simulink model "PMSM_FOC_Tractio"  (R2019b)
settings: Solver=FixedStepAuto  StartTime=0.0  StopTime=10  RelTol=1e-3
model workspace (MAT data in the model file):
  wc : Simulink.Parameter (value not decoded)
values from neighbouring files (symbols this model uses):
  CL_Param = tmp_CL_Param    [PMSM_Parameters.m]
  Cosine_table = [1,0.999995293095708,0.999990587122738,0.999985881149769,0.999981174245477,0.999967055395246,0.999952936545014,0.999938818626106,0.999924698844552,0.999901168979704,0.999877639114857,0.999854108318687,0.999830577522516,0.999797635711730,0.999764694832265,0.999731753021479,0.999698810279369,0.999656459316611,0.999614108353853,0.999571758322418,0.999529405497015,0.999477646313608,0.999425887130201,0 ...(+75635 chars)    [Motor_Table.m]
  ctrlParamsPI = tmp_ctrlParamsPI    [PMSM_Parameters.m]
  Flux_weak = tmp_Fluxweak_struct    [PMSM_Parameters.m]
  Hall_Parameter = tmp_Hall_struct    [PMSM_Parameters.m]
  HFI = tmp_HFI_struct    [PMSM_Parameters.m]
  inverter = struct    [PMSM_Parameters.m]
  MTPA_id_table = [-1.39452500000000,-1.36697494250000,-1.33970177000000,-1.31270548250000,-1.28598608000000,-1.25954356250000,-1.23337793000000,-1.20748918250000,-1.18187732000000,-1.15654234250000,-1.13148425000000,-1.10670304250000,-1.08219872000000,-1.05797128250000,-1.03402073000000,-1.01034706250000,-0.986950280000000,-0.963830382500000,-0.940987370000000,-0.918421242500000,-0.896132000000000,-0.8741196425000 ...(+3439 chars)    [Motor_Table.m]
  MTPA_iq_table = [-10.2740250000000,-10.1791705677750,-10.0840783722000,-9.98875081492500,-9.89319029760000,-9.79739922187500,-9.70137998940000,-9.60513500182500,-9.50866666080000,-9.41197736797500,-9.31506952500000,-9.21794553352500,-9.12060779520000,-9.02305871167500,-8.92530068460000,-8.82733611562500,-8.72916740640000,-8.63079695857500,-8.53222717380000,-8.43346045372500,-8.33449920000000,-8.23534581427500,-8. ...(+3121 chars)    [Motor_Table.m]
  MTPA_Te_Max = single(1.50)    [Motor_Table.m]
  MTPA_Te_Min = single(-1.50)    [Motor_Table.m]
  OPL_Param = tmp_OPL_Param    [PMSM_Parameters.m]
  pmsm = struct    [PMSM_Parameters.m]
  Resolver_Parameter = tmp_Resolver_struct    [PMSM_Parameters.m]
  Sine_table = [0,0.00153398793190718,0.00306797679513693,0.00460196565836668,0.00613595545291901,0.00766988657414913,0.00920381769537926,0.0107377488166094,0.0122716808691621,0.0138054965063930,0.0153393121436238,0.0168731296434999,0.0184069443494082,0.0199405867606401,0.0214742291718721,0.0230078706517816,0.0245415139943361,0.0260749254375696,0.0276083368808031,0.0291417483240366,0.0306751597672701,0.032208281 ...(+75648 chars)    [Motor_Table.m]
  SMO = temp_SMO    [PMSM_Parameters.m]
undefined symbols (not defined in the file or in its folder): DiscIntNeverNeededParam, Kiv, Kiw, Kpv, Kpw, magnitude, sigbuilder_block, SVPWM, Vdc
libraries: powerlib x29, fl_lib x18, simulink x10, nesl_utility x7, eeGeneralControl x4, dspstat3 x3, eeDiscretePi x2, powerlib_extras x1, ee_lib x1
(part 3 of 6)

== system PMSM_FOC_Tractio/Motor_Control/Motor_Control_Funtion/Angle_Speed_100us/Speed_Angle_Selector ==
  Resolver_Speed : Inport
  Resolver_Angle : Inport  Port=2
  Resolver_PLL_Speed : Inport  Port=3
  Resolver_PLL_Angle : Inport  Port=4
  Sensorless_Speed : Inport  Port=5
  Sensorless_Angle : Inport  Port=6
  Hall_Speed : Inport  Port=7
  Hall_Angle : Inport  Port=8
  Hall : Subsystem
  Hall_Angle_Enable : Constant  Value=Hall_Parameter.Angle_Enable  OutDataTypeStr=uint8
  If{1..3,5} (4 alike) : If  IfExpression=u1==1  ShowElse=off
  Merge : Merge  Inputs=4
  Merge1 : Merge  Inputs=4
  Resolver_Dir : Subsystem
  Resolver_Enable : Constant  Value=Resolver_Parameter.Angle_Enable  OutDataTypeStr=uint8
  Resolver_PLL : Subsystem
  Resolver_PLL_Enable : Constant  Value=Resolver_Parameter.PLL_Angle_Enable  OutDataTypeStr=uint8
  Sensorless : Subsystem
  Sensorless_Enable : Constant  Value=OPL_Param.Func_Enable  OutDataTypeStr=uint8
  Speed : Outport
  Theta : Outport  Port=2
  wires:
  If5/1 -> Resolver_Dir/Action
  Resolver_Enable/1 -> If5/1
  Hall_Speed/1 -> Hall/1(In1)
  Hall_Angle/1 -> Hall/2(In2)
  Sensorless_Speed/1 -> Sensorless/1(In1)
  Sensorless_Angle/1 -> Sensorless/2(In2)
  Resolver_Speed/1 -> Resolver_Dir/1(In1)
  Resolver_Angle/1 -> Resolver_Dir/2(In2)
  Resolver_PLL_Speed/1 -> Resolver_PLL/1(In1)
  Resolver_PLL_Angle/1 -> Resolver_PLL/2(In2)
  If1/1 -> Resolver_PLL/Action
  Resolver_PLL_Enable/1 -> If1/1
  Sensorless_Enable/1 -> If2/1
  If2/1 -> Sensorless/Action
  Hall_Angle_Enable/1 -> If3/1
  If3/1 -> Hall/Action
  Resolver_Dir/1(Out1) -> Merge/1
  Resolver_PLL/1(Out1) -> Merge/2
  Sensorless/1(Out1) -> Merge/3
  Hall/1(Out1) -> Merge/4
  Resolver_Dir/2(Out2) -> Merge1/1
  Resolver_PLL/2(Out2) -> Merge1/2
  Sensorless/2(Out2) -> Merge1/3
  Hall/2(Out2) -> Merge1/4
  Merge1/1 -> Theta/1
  Merge/1 -> Speed/1

== system PMSM_FOC_Tractio/Motor_Control/Motor_Control_Funtion/Angle_Speed_100us/Speed_Resolver ==
  Theta : Inport
  Action Port : ActionPort  ActionPortLabel=if(u1==1)
  DT2 : DataTypeConversion  OutDataTypeStr=single
  Scope : Scope
  Scope1 : Scope
  Speed_cacl : Subsystem  TreatAsAtomicUnit=on
      settings: RTWSystemCode=Nonreusable function  RTWFcnNameOpts=Use subsystem name
  Speed_out : Outport
  Dir_Angle : Outport  Port=2
  wires:
  Theta/1 -> DT2/1, Speed_cacl/1(position)  "Theta_input"
  Speed_cacl/1(Speed_RPM) -> Scope1/1, Speed_out/1  "Speed_RPM_Filtered"
  DT2/1 -> Scope/1, Dir_Angle/1  "Direct_Angle"

== system PMSM_FOC_Tractio/Motor_Control/Motor_Control_Funtion/Angle_Speed_100us/Startup_OPL ==
  OPL_Torque : Inport
  OPL_State : Inport  Port=2
  Smo_theta : Inport  Port=3
  Action Port : ActionPort  ActionPortLabel=if(u1==2|u1==3 | u1==3)
  If2 : If  IfExpression=u1==2  ElseIfExpressions=u1==3  ShowElse=off
  Merge : Merge
  Merge1 : Merge
  OPL_SpeedRPM : Constant  Value=OPL_Param.Target_RPM
  Scope3 : Scope  NumInputPorts=3
  Subsystem : Subsystem
  Subsystem1 : Subsystem
  Force_Angle : Outport
  OPL_Torque_Com : Outport  Port=2
  wires:
  OPL_State/1 -> If2/1
  If2/1 -> Subsystem/Action
  OPL_Torque/1 -> Subsystem1/1(OPL_Torque), Subsystem/2(OPL_Torque)
  If2/2 -> Subsystem1/Action
  Subsystem/1(Force_Angle) -> Merge/1
  Subsystem1/1(Force_Angle) -> Merge/2
  Merge/1 -> Force_Angle/1  "FOC_Angle"
  Subsystem/2(OPL_Torque_Com) -> Merge1/1
  Subsystem1/2(OPL_Torque_Com) -> Merge1/2
  Merge1/1 -> OPL_Torque_Com/1  "FOC_Angle"
  OPL_SpeedRPM/1 -> Subsystem1/3(Force_RPM), Subsystem/1(OPL_Speed)
  Smo_theta/1 -> Scope3/2, Subsystem/3(Smo_theta)
  Subsystem/3(Delta_theta) -> Subsystem1/2(Delta_theta)
  Subsystem/4(Force_Switch) -> Scope3/3, Subsystem1/4(Force_Switch)
  Subsystem1/3(Force_Angle1) -> Scope3/1

== system PMSM_FOC_Tractio/Motor_Control/Motor_Control_Funtion/Angle_Speed_100us/Subsystem ==
  Action Port : ActionPort  ActionPortLabel=if((u1==1)&(u2==1))
  Sensorless_Enable : Constant  OutDataTypeStr=boolean
  Out1 : Outport
  wires:
  Sensorless_Enable/1 -> Out1/1

== system PMSM_FOC_Tractio/Motor_Control/Motor_Control_Funtion/Angle_Speed_100us/Subsystem1 ==
  Action Port : ActionPort  ActionPortLabel=else
  Sensorless_Disable : Constant  Value=0  OutDataTypeStr=boolean
  Out1 : Outport
  wires:
  Sensorless_Disable/1 -> Out1/1

== system PMSM_FOC_Tractio/Motor_Control/Motor_Control_Funtion/Control_Command_2ms/Speed_PI ==
  Speed_Command : Inport
  Speed_Measured : Inport  Port=2
  HFI_State : Inport  Port=3
  Motor_State : Inport  Port=4
  BLDC_State : Inport  Port=5
  Action Port : ActionPort  ActionPortLabel=case [ 1 ]:
  Add2 : Sum  Inputs=|+-
  Hall_Enalble : Constant  Value=Hall_Parameter.BLDC_Start  OutDataTypeStr=uint8
  If1 : If  NumInputs=2  IfExpression=(u1==1)&(u2==3)|(u1~=1)  ShowElse=off
  Scope2 : Scope
  Speed_PI : Subsystem
  Iq_ref : Outport  VectorParamsAs1DForOutWhenUnconnected=off
  wires:
  Speed_Command/1 -> Add2/1
  Speed_Measured/1 -> Add2/2
  Add2/1 -> Speed_PI/1(PI_input)  "currentControlError"
  Speed_PI/1(PI_out) -> Iq_ref/1, Scope2/1
  HFI_State/1 -> Speed_PI/2(HFI_State)
  Motor_State/1 -> Speed_PI/3(Motor_State)
  BLDC_State/1 -> If1/2
  Hall_Enalble/1 -> If1/1
  If1/1 -> Speed_PI/Action

== system PMSM_FOC_Tractio/Motor_Control/Motor_Control_Funtion/Control_Command_2ms/Switch Case Action Subsystem ==
  Iq_in : Inport
  Action Port : ActionPort  ActionPortLabel=case [ 2 ]:
  Iq_out : Outport
  wires:
  Iq_in/1 -> Iq_out/1

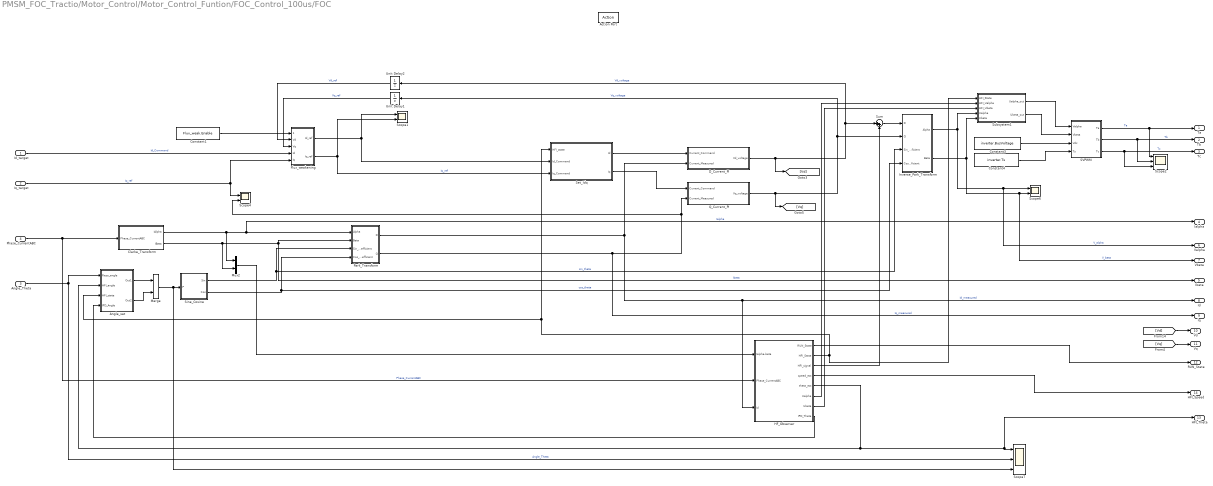
== system PMSM_FOC_Tractio/Motor_Control/Motor_Control_Funtion/FOC_Control_100us/FOC ==
  Id_target : Inport
  Iq_target : Inport  Port=2
  Angle_Theta : Inport  Port=3  OutMin=0  OutMax=2*pi
  Phase_CurrentABC : Inport  Port=4  PortDimensions=3
  Action Port : ActionPort  ActionPortLabel=if((u1==1)&(u2==3)|(u1~=1))
  Angle_set : Subsystem  TreatAsAtomicUnit=on
      settings: RTWSystemCode=Nonreusable function  RTWFcnNameOpts=Use subsystem name
  Clarke_Transform : Subsystem  TreatAsAtomicUnit=on
      settings: RTWSystemCode=Nonreusable function  RTWFcnNameOpts=Use subsystem name
  Constant1 : Constant  Value=Flux_weak.Enable  OutDataTypeStr=single
  Constant3 : Constant  Value=inverter.BusVoltage  OutDataTypeStr=single
  Constant4 : Constant  Value=inverter.Ts  OutDataTypeStr=single
  D_Current_PI : Subsystem  TreatAsAtomicUnit=on
      settings: RTWSystemCode=Nonreusable function  RTWFcnNameOpts=Use subsystem name
  "Flux_weakening " : Subsystem
  HF_Observer : Subsystem  TreatAsAtomicUnit=on
      settings: RTWSystemCode=Nonreusable function  RTWFcnNameOpts=Use subsystem name  RTWFileNameOpts=Use subsystem name
  Inverse_Park_Transform : Subsystem  TreatAsAtomicUnit=on
      settings: RTWSystemCode=Nonreusable function  RTWFcnNameOpts=Use subsystem name
      mask Display:
      | port_label('input',1,'D')
      | port_label('input',2,'Q')
      | port_label('input',3,'Sin')
      | port_label('input',4,'Cos')
      | port_label('output',1,'\alpha','texmode', 'on')
      | port_label('output',2,'\beta','texmode', 'on')
  Merge : Merge
  Mux2 : Mux  Inputs=2
  Park_Transform : Subsystem  TreatAsAtomicUnit=on
      settings: RTWSystemCode=Nonreusable function  RTWFcnNameOpts=Use subsystem name
      mask Display:
      | port_label('input',1,'\alpha','texmode', 'on')
      | port_label('input',2,'\beta','texmode', 'on')
      | port_label('input',3,'Sin')
      | port_label('input',4,'Cos')
      | port_label('output',1,'D')
      | port_label('output',2,'Q')
  Q_Current_PI : Subsystem  TreatAsAtomicUnit=on
      settings: RTWSystemCode=Nonreusable function  RTWFcnNameOpts=Use subsystem name
  SVPWM : Subsystem  AncestorBlock=SVPWM/SVPWM  TreatAsAtomicUnit=on  RTWFcnName=SVPWM  RTWFileName=SVPWM
      settings: RTWSystemCode=Nonreusable function  RTWFcnNameOpts=Use subsystem name
      mask Display:
      | plot([0.000 0.020 0.041 0.061 0.082 0.102 0.122 0.143 0.163 0.184 0.204 0.224 0.245 0.265 0.286 0.306 0.327 0.347 0.367 0.388 0.408 0.429 0.449 0.469 0.490 0.510 0.531 0.551 0.571 0.592 0.612 0.633 0.653 0.673 0.694 0.714 0.735 0.755 0.776 0.796 0.816 0.837 0.857 0.878 0.898 0.918 0.939 0.959 0.980 1.000 ], ...
      |      [0.500 0.586 0.671 0.753 0.831 0.858 0.875 0.885 0.890 0.887 0.879 0.864 0.844 0.855 0.872 0.884 0.889 0.888 0.881 0.867 0.847 0.793 0.713 0.629 0.543 0.457 0.371 0.287 0.207 0.153 0.133 0.119 0.112 0.111 0.116 0.128 0.145 0.156 0.136 0.121 0.113 0.110 0.115 0.125 0.142 0.169 0.247 0.329 0.414 0.500 ])
  Scope1 : Scope  NumInputPorts=2
  Scope2 : Scope  NumInputPorts=3
  Scope4 : Scope  NumInputPorts=2
  Scope6 : Scope  NumInputPorts=2
  Scope7 : Scope  NumInputPorts=3
  Set_Idq : Subsystem  TreatAsAtomicUnit=on
      settings: RTWSystemCode=Nonreusable function  RTWFcnNameOpts=Use subsystem name
  Sine_Cosine : Subsystem  TreatAsAtomicUnit=on
      settings: RTWSystemCode=Nonreusable function  RTWFcnNameOpts=Use subsystem name
  Subsystem1 : Subsystem
  Sum : Sum  Inputs=|++
  Unit Delay1 : UnitDelay  SampleTime=-1  HasFrameUpgradeWarning=on
  Unit Delay2 : UnitDelay  SampleTime=-1  HasFrameUpgradeWarning=on
  Ta : Outport
  Tb : Outport  Port=2
  Tc : Outport  Port=3
  Ialpha : Outport  Port=4
  Ibeta : Outport  Port=5
  Valpha : Outport  Port=6
  Vbeta : Outport  Port=7
  Id : Outport  Port=8
  Iq : Outport  Port=9
  Vd : Outport  Port=10
  Vq : Outport  Port=11
  RUN_State : Outport  Port=12
  HFI_Theta : Outport  Port=13
  HFI_Speed : Outport  Port=14
  wires:
  Park_Transform/1(D) -> HF_Observer/3(Id), Id/1, D_Current_PI/2(Current_Measured)  "Id_measured"
  Constant4/1 -> SVPWM/4(Ts)
  SVPWM/3(Tc) -> Tc/1, Scope2/3  "Tc"
  SVPWM/2(Tb) -> Scope2/2, Tb/1  "Tb"
  Park_Transform/2(Q) -> Iq/1, Scope4/2, Q_Current_PI/2(Current_Measured)  "Iq_measured"
  Sine_Cosine/2(Cos) -> Park_Transform/4(Cos_Coefficient), Inverse_Park_Transform/4(Cos_Coefficient)  "cos_theta"
  Sine_Cosine/1(Sin) -> Park_Transform/3(Sin_Coefficient), Inverse_Park_Transform/3(Sin_Coefficient)  "sin_theta"
  Constant3/1 -> SVPWM/3(Vdc)
  D_Current_PI/1(Vd_voltage) -> [Vd], Unit Delay2/1, Sum/1  "Vd_voltage"
  Q_Current_PI/1(Vq_voltage) -> [Vq], Unit Delay1/1, Inverse_Park_Transform/2(Q)  "Vq_voltage"
  SVPWM/1(Ta) -> Scope2/1, Ta/1  "Ta"
  Id_target/1 -> "Flux_weakening "/4(Id)  "Id_Command"
  Iq_target/1 -> "Flux_weakening "/5(Iq), Scope4/1  "Iq_ref"
  Clarke_Transform/2(IBeta) -> Mux2/2, Ibeta/1, Park_Transform/2(Beta)  "Ibeta"
  Clarke_Transform/1(IAlpha) -> Ialpha/1, Park_Transform/1(Alpha), Mux2/1  "Ialpha"
  Unit Delay2/1 -> "Flux_weakening "/2(Vd)  "Vd_ref"
  Unit Delay1/1 -> "Flux_weakening "/3(Vq)  "Vq_ref"
  "Flux_weakening "/1(Id_ref) -> Scope1/1, Set_Idq/2(Id_Command)
  "Flux_weakening "/2(Iq_ref) -> Set_Idq/3(Iq_Command), Scope1/2  "Iq_ref"
  Constant1/1 -> "Flux_weakening "/1(Enable)
  Inverse_Park_Transform/1(Alpha) -> Scope6/1, Valpha/1, Subsystem1/4(Ualpha)  "V_alpha"
  Inverse_Park_Transform/2(Beta) -> Scope6/2, Vbeta/1, Subsystem1/5(Ubeta)  "V_beta"
  Phase_CurrentABC/1 -> HF_Observer/2(Phase_CurrentABC), Clarke_Transform/1(Phase_CurrentABC)  "Phase_CurrentABC"
  Sum/1 -> Inverse_Park_Transform/1(D)
  HF_Observer/3(HFI_signal) -> Sum/2
  HF_Observer/4(speed_est) -> HFI_Speed/1
  Angle_Theta/1 -> Scope7/2, Angle_set/1(Reso_angle)  "Angle_Theta"
  Mux2/1 -> HF_Observer/1(Ialpha-beta)
  HF_Observer/5(theta_est) -> HFI_Theta/1, Scope7/1, Angle_set/2(HFI_angle)
  Merge/1 -> Scope7/3, Sine_Cosine/1(P)
  Angle_set/1(Out1) -> Merge/1
  Angle_set/2(Out2) -> Merge/2
  Subsystem1/1(Ualpha_out) -> SVPWM/1(Valpha)
  Subsystem1/2(Ubeta_out) -> SVPWM/2(Vbeta)
  HF_Observer/6(Ualpha) -> Subsystem1/2(HFI_Ualpha)
  HF_Observer/7(Ubeta) -> Subsystem1/3(HFI_Ubeta)
  HF_Observer/2(HFI_State) -> Subsystem1/1(HFI_State), Set_Idq/1(HFI_state), Angle_set/3(HFI_state)
  HF_Observer/1(RUN_State) -> RUN_State/1
  Set_Idq/1(Id) -> D_Current_PI/1(Current_Command)
  Set_Idq/2(Iq) -> Q_Current_PI/1(Current_Command)
  HF_Observer/8(IPD_Theta) -> Angle_set/4(IPD_Angle)
  [Vq] -> Vq/1
  [Vd] -> Vd/1

== system PMSM_FOC_Tractio/Motor_Control/Motor_Control_Funtion/FOC_Control_100us/Iq_selector ==
  Motor_state : Inport
  PI_IQ : Inport  Port=2
  OPL_IQ : Inport  Port=3
  If1 : If  IfExpression=u1 ==2 | u1 ==3
  Merge : Merge
  Subsystem : Subsystem
  Subsystem1 : Subsystem
  Iq_ref : Outport
  wires:
  Motor_state/1 -> If1/1
  If1/1 -> Subsystem/Action
  OPL_IQ/1 -> Subsystem/1(In1)
  PI_IQ/1 -> Subsystem1/1(In1)
  Subsystem/1(Out1) -> Merge/1
  Subsystem1/1(Out1) -> Merge/2
  Merge/1 -> Iq_ref/1
  If1/2 -> Subsystem1/Action

== system PMSM_FOC_Tractio/Motor_Control/Motor_Control_Funtion/FOC_Control_100us/MTPA ==
  Te_ref : Inport
  1-D Lookup Table4 : Lookup_n-D  NumberOfTableDimensions=1  LookupTableObject=''  BreakpointsForDimension1=single(linspace(MTPA_Te_Min,MTPA_Te_Max,length(MTPA_id_table)));  BreakpointsForDimension1FirstPoint=10  BreakpointsForDimension2FirstPoint=10  BreakpointsForDimension1Spacing=12  BreakpointsForDimension2Spacing=12  IndexSearchMethod=Evenly spaced points  Table=MTPA_id_table  InterpMethod=Flat  DiagnosticForOutOfRangeInput=Error  InternalRulePriority=Speed  RndMeth=Simplest  InputSameDT=on
  1-D Lookup Table5 : Lookup_n-D  NumberOfTableDimensions=1  LookupTableObject=''  BreakpointsForDimension1=single(linspace(MTPA_Te_Min,MTPA_Te_Max,length(MTPA_id_table)));  BreakpointsForDimension1FirstPoint=10  BreakpointsForDimension2FirstPoint=10  BreakpointsForDimension1Spacing=12  BreakpointsForDimension2Spacing=12  IndexSearchMethod=Evenly spaced points  Table=MTPA_iq_table  InterpMethod=Flat  DiagnosticForOutOfRangeInput=Error  InternalRulePriority=Speed  RndMeth=Simplest  InputSameDT=on
  Saturation : Saturate  UpperLimit=MTPA_Te_Max-0.01  LowerLimit=MTPA_Te_Min+0.01
  Saturation1 : Saturate  UpperLimit=MTPA_Te_Max-0.01  LowerLimit=MTPA_Te_Min+0.01
  Id_ref : Outport
  Iq_ref : Outport  Port=2
  wires:
  Te_ref/1 -> Saturation1/1, Saturation/1
  Saturation/1 -> 1-D Lookup Table4/1
  Saturation1/1 -> 1-D Lookup Table5/1
  1-D Lookup Table4/1 -> Id_ref/1
  1-D Lookup Table5/1 -> Iq_ref/1

== system PMSM_FOC_Tractio/Motor_Control/Motor_Control_Funtion/Motor_State_10ms/Power_Cacl ==
  Id : Inport
  Vd : Inport  Port=2
  Iq : Inport  Port=3
  Vq : Inport  Port=4
  Add : Sum
  Product : Product
  Product1 : Product
  Power : Outport
  wires:
  Id/1 -> Product/1
  Vd/1 -> Product/2
  Iq/1 -> Product1/1
  Vq/1 -> Product1/2
  Product/1 -> Add/1
  Product1/1 -> Add/2
  Add/1 -> Power/1

== system PMSM_FOC_Tractio/Motor_Control/Motor_Control_Funtion/Motor_State_10ms/Torque_Cacl ==
  Id : Inport
  Iq : Inport  Port=2
  Constant : Constant  Value=3/2  OutDataTypeStr=single
  Constant1 : Constant  Value=pmsm.PolePairs  OutDataTypeStr=single
  Constant2 : Constant  Value=pmsm.FluxLinkage  OutDataTypeStr=single
  Constant3 : Constant  Value=pmsm.InductanceLd  OutDataTypeStr=single
  Constant4 : Constant  Value=pmsm.InductanceLq  OutDataTypeStr=single
  Product{,1..4} (5 alike) : Product
  Subtract : Sum
  Subtract1 : Sum  Inputs=+-
  Torque : Outport
  wires:
  Constant1/1 -> Product/1
  Constant/1 -> Product/2
  Constant2/1 -> Product1/1
  Iq/1 -> Product1/2, Product3/1
  Product1/1 -> Subtract/1
  Constant3/1 -> Subtract1/1
  Constant4/1 -> Subtract1/2
  Subtract1/1 -> Product2/1
  Id/1 -> Product2/2
  Product2/1 -> Product3/2
  Product3/1 -> Subtract/2
  Product/1 -> Product4/1
  Subtract/1 -> Product4/2
  Product4/1 -> Torque/1

== system PMSM_FOC_Tractio/PMSM/Control/Control/Commutation ==
  Hall : Inport
  Bias : Bias  Bias=-1
  Bit concatenate : Subsystem
  Data Type Conversion : DataTypeConversion
  Direct Lookup Table (n-D)2 : LookupNDDirect  InputsSelectThisObjectFromTable=Vector  Table=[0 0 0 1 1 0;0 1 1 0 0 0;0 1 0 0 0 1;1 0 0 0 1 0;1 0 1 0 0 0;0 0 0 1 0 1]
  S : Outport  VectorParamsAs1DForOutWhenUnconnected=off
  wires:
  Hall/1 -> Bit concatenate/1(u)
  Bit concatenate/1(y) -> Data Type Conversion/1
  Direct Lookup Table (n-D)2/1 -> S/1
  Data Type Conversion/1 -> Bias/1
  Bias/1 -> Direct Lookup Table (n-D)2/1

== system PMSM_FOC_Tractio/PMSM/SpeedAndAngle/ACC_OMG/Six_point ==
  In1 : Inport
  Merge2 : Merge  Inputs=6
  Scope : Scope  NumInputPorts=2
  Sector_1 : Subsystem
  Sector_2 : Subsystem
  Sector_3 : Subsystem
  Sector_4 : Subsystem
  Sector_5 : Subsystem
  Sector_6 : Subsystem
  Switch Case2 : SwitchCase  CaseConditions={1,2,3,4,5,6}  ShowDefaultCase=off
  Out1 : Outport
  wires:
  Sector_4/1(Angle_0) -> Merge2/4
  Switch Case2/5 -> Sector_5/Action
  Sector_6/1(Angle_0) -> Merge2/6
  Sector_5/1(Angle_0) -> Merge2/5
  Switch Case2/6 -> Sector_6/Action
  Switch Case2/3 -> Sector_3/Action
  Switch Case2/4 -> Sector_4/Action
  Sector_1/1(Angle_0) -> Merge2/1
  Switch Case2/2 -> Sector_2/Action
  In1/1 -> Scope/1, Switch Case2/1
  Sector_3/1(Angle_0) -> Merge2/3
  Switch Case2/1 -> Sector_1/Action
  Sector_2/1(Angle_0) -> Merge2/2
  Merge2/1 -> Scope/2, Out1/1

== system PMSM_FOC_Tractio/PMSM/SpeedAndAngle/ADC_IRQ/HallAngle_calibration ==
  Angle_input : Inport
  Angle_offset : Constant  Value=SMO.Angle_offset
  If Action Subsystem1 : Subsystem  TreatAsAtomicUnit=on
  If Action Subsystem2 : Subsystem  TreatAsAtomicUnit=on
  If Action Subsystem3 : Subsystem  TreatAsAtomicUnit=on
  If1 : If  IfExpression=u1 > 6.283185307  ElseIfExpressions=u1<0
  Merge1 : Merge  Inputs=3
  Subtract1 : Sum
  Angle_output : Outport
  wires:
  Angle_input/1 -> Subtract1/1
  Angle_offset/1 -> Subtract1/2  "Control_ModeCommand"
  If1/1 -> If Action Subsystem2/Action
  If1/3 -> If Action Subsystem1/Action
  If Action Subsystem2/1(Out1) -> Merge1/1
  Subtract1/1 -> If Action Subsystem3/1(In1), If Action Subsystem1/1(In1), If Action Subsystem2/1(In1), If1/1
  If Action Subsystem1/1(Out1) -> Merge1/3
  If Action Subsystem3/1(Out1) -> Merge1/2
  If1/2 -> If Action Subsystem3/Action
  Merge1/1 -> Angle_output/1

== system PMSM_FOC_Tractio/Motor_Control/Motor_Control_Funtion/Angle_Speed_100us/Angle_Selector/Subsystem ==
  In1 : Inport
  Action Port : ActionPort  ActionPortLabel=if(u1 ==2 | u1 ==3)
  Out1 : Outport
  wires:
  In1/1 -> Out1/1

== system PMSM_FOC_Tractio/Motor_Control/Motor_Control_Funtion/Angle_Speed_100us/Angle_Selector/Subsystem1 ==
  In1 : Inport
  Action Port : ActionPort  ActionPortLabel=elseif(u1 ==4)
  Out1 : Outport
  wires:
  In1/1 -> Out1/1

== system PMSM_FOC_Tractio/Motor_Control/Motor_Control_Funtion/Angle_Speed_100us/Resolver_Observer/Angle_calibration ==
  Angle_input : Inport
  Angle_offset : Constant  Value=Resolver_Parameter.PLL_Angle_offset
  If Action Subsystem1 : Subsystem  TreatAsAtomicUnit=on
  If Action Subsystem2 : Subsystem  TreatAsAtomicUnit=on
  If Action Subsystem3 : Subsystem  TreatAsAtomicUnit=on
  If1 : If  IfExpression=u1 > 6.283185307  ElseIfExpressions=u1<0
  Merge1 : Merge  Inputs=3
  Subtract1 : Sum
  Angle_output : Outport
  wires:
  If1/2 -> If Action Subsystem3/Action
  If Action Subsystem1/1(Out1) -> Merge1/3
  If1/3 -> If Action Subsystem1/Action
  If Action Subsystem3/1(Out1) -> Merge1/2
  If Action Subsystem2/1(Out1) -> Merge1/1
  Subtract1/1 -> If Action Subsystem3/1(In1), If Action Subsystem1/1(In1), If Action Subsystem2/1(In1), If1/1
  If1/1 -> If Action Subsystem2/Action
  Angle_offset/1 -> Subtract1/2
  Angle_input/1 -> Subtract1/1
  Merge1/1 -> Angle_output/1

== system PMSM_FOC_Tractio/Motor_Control/Motor_Control_Funtion/Angle_Speed_100us/Resolver_Observer/Resolver_Angle_cacl ==
  Sin_Cos : Inport
  2*pi : Constant  Value=2*pi  OutDataTypeStr=single  SampleTime=-1
  B : Selector  IndexMode=Zero-based  InputPortWidth=2  IndexOptions=Index vector (dialog)  Indices=0  OutputSizes=1
  C : Selector  IndexMode=Zero-based  InputPortWidth=2  IndexOptions=Index vector (dialog)  Indices=1  OutputSizes=1
  Constant : Constant  OutDataTypeStr=single  SampleTime=-1
  Discrete-Time Integrator : DiscreteIntegrator  SampleTime=-1  ICPrevOutput=DiscIntNeverNeededParam  ICPrevScaledInput=DiscIntNeverNeededParam
  Gain : Gain  Gain=15/(2*pi)
  LPF : DiscreteFilter  Numerator=[0 0.04]  Denominator=[1 -0.96]
  Math Function : Math  Operator=mod  SaturateOnIntegerOverflow=on
  PID Controller : simulink/Continuous/PID Controller  Controller=PI  Form=Parallel  TimeDomain=Discrete-time  SampleTime=-1  IntegratorMethod=Forward Euler  FilterMethod=Forward Euler  ControllerParametersSource=internal  P=141  I=10000  D=0  UseFilter=off  N=100  TunerSelectOption=Transfer Function Based (PID Tuner App)  InitialConditionSource=internal  InitialConditionForIntegrator=0  InitialConditionForFilter=0  DifferentiatorICPrevScaledInput=0  ExternalReset=none  TrackingMode=off  Kt=1  LimitOutput=off  UpperSaturationLimit=inf  LowerSaturationLimit=-inf  LinearizeAsGain=on  AntiWindupMode=none  Kb=1  POutMin=[]  POutMax=[]  IOutMin=[]  IOutMax=[]  DOutMin=[]  DOutMax=[]  NOutMin=[]  NOutMax=[]  SumOutMin=[]  SumOutMax=[]  SaturationOutMin=[]  SaturationOutMax=[]  PParamMin=[]  PParamMax=[]  IParamMin=[]  IParamMax=[]  DParamMin=[]  DParamMax=[]  NParamMin=[]  NParamMax=[]  KbParamMin=[]  KbParamMax=[]  KtParamMin=[]  KtParamMax=[]  KbOutMin=[]  KbOutMax=[]  KtOutMin=[]  KtOutMax=[]  IntegratorOutMin=[]  IntegratorOutMax=[]  FilterOutMin=[]  FilterOutMax=[]  SumI1OutMin=[]  SumI1OutMax=[]  SumI2OutMin=[]  SumI2OutMax=[]  SumI3OutMin=[]  SumI3OutMax=[]  SumI4OutMin=[]  SumI4OutMax=[]  SumDOutMin=[]  SumDOutMax=[]  DifferentiatorOutMin=[]  DifferentiatorOutMax=[]  FilterDiffOutCoefMin=[]  FilterDiffOutCoefMax=[]  ReciprocalOutMin=[]  ReciprocalOutMax=[]  SumDenOutMin=[]  SumDenOutMax=[]  SumNumOutMin=[]  SumNumOutMax=[]  DivideOutMin=[]  DivideOutMax=[]  IntegratorContinuousStateAttributes=''  IntegratorStateMustResolveToSignalObject=off  IntegratorRTWStateStorageClass=Auto  FilterContinuousStateAttributes=''  FilterStateMustResolveToSignalObject=off  FilterRTWStateStorageClass=Auto  ParallelPVariant=InternalParameters  IdealPVariant=Disabled  IVariant=InternalParameters  DVariant=Disabled  IntegratorVariant=Discrete  SatVariant=Disabled  AWVariant=Passthrough  PCopyVariant=Disabled  TRVariant=Disabled  FdbkBlocksVariant=Forward  IdealPFdbkVariant=Disabled  SatFdbkVariant=Disabled  DerivativeFilterVariant=Disabled  NVariant=Disabled  NCopyVariant=Disabled_SignalSpec  FilterICVariant=Disabled  IntegratorICVariant=InternalICs  ExternalResetVariant=Disabled  TRSumVariant=Passthrough  SumFdbkVariant=Disabled  SumVariant=Sum_PI
  Product : Product  OutDataTypeStr=single
  Product{1..4} (4 alike) : Product
  Scope : Scope  NumInputPorts=2
  Scope{1,3..4,6..7} (5 alike) : Scope
  Scope2 : Scope  NumInputPorts=2
  Scope5 : Scope  NumInputPorts=2
  Sine_Cosine : Subsystem  TreatAsAtomicUnit=on
      settings: RTWSystemCode=Nonreusable function  RTWFcnNameOpts=Use subsystem name
  Sum1 : Sum  Inputs=-+
  Unit Delay4 : UnitDelay  SampleTime=-1  HasFrameUpgradeWarning=on
  constant : Constant  OutDataTypeStr=single
  "pole pairs " : Gain  OutDataTypeStr=single
  Velocity : Outport  VectorParamsAs1DForOutWhenUnconnected=off
  Angle : Outport  Port=2  VectorParamsAs1DForOutWhenUnconnected=off
  wires:
  Product2/1 -> Scope2/2, Product4/1
  Product4/1 -> Scope/2, Sum1/2
  Sin_Cos/1 -> C/1, B/1
  Unit Delay4/1 -> Product/2
  Sum1/1 -> PID Controller/1
  Product3/1 -> Scope/1, Sum1/1
  Constant/1 -> Product/1
  constant/1 -> Product2/1, Product1/1
  Product/1 -> Sine_Cosine/1(P)
  Sine_Cosine/1(Sin) -> Product1/2
  Product1/1 -> Scope2/1, Product3/2
  Math Function/1 -> Unit Delay4/1, Angle/1, Scope4/1  "Angle_Theta"
  Gain/1 -> LPF/1, Scope3/1  "Speed_RPM"
  Discrete-Time Integrator/1 -> Scope6/1, "pole pairs "/1
  "pole pairs "/1 -> Math Function/1
  PID Controller/1 -> Discrete-Time Integrator/1, Gain/1
  2*pi/1 -> Math Function/2
  B/1 -> Scope1/1, Product3/1, Scope5/2, Scope5/1  "Vx"
  C/1 -> Product4/2, Scope7/1  "Vy"
  LPF/1 -> Velocity/1
  Sine_Cosine/2(Cos) -> Product2/2

== system PMSM_FOC_Tractio/Motor_Control/Motor_Control_Funtion/Angle_Speed_100us/SMO/Angle_calibration ==
  Angle_input : Inport
  Angle_offset : Constant  Value=SMO.Angle_offset
  If Action Subsystem1 : Subsystem  TreatAsAtomicUnit=on
  If Action Subsystem2 : Subsystem  TreatAsAtomicUnit=on
  If Action Subsystem3 : Subsystem  TreatAsAtomicUnit=on
  If1 : If  IfExpression=u1 > 6.283185307  ElseIfExpressions=u1<0
  Merge1 : Merge  Inputs=3
  Subtract1 : Sum
  Angle_output : Outport
  wires:
  Angle_input/1 -> Subtract1/1
  Angle_offset/1 -> Subtract1/2  "Control_ModeCommand"
  If1/1 -> If Action Subsystem2/Action
  If1/3 -> If Action Subsystem1/Action
  If Action Subsystem2/1(Out1) -> Merge1/1
  Subtract1/1 -> If Action Subsystem3/1(In1), If Action Subsystem1/1(In1), If Action Subsystem2/1(In1), If1/1
  If Action Subsystem1/1(Out1) -> Merge1/3
  If Action Subsystem3/1(Out1) -> Merge1/2
  If1/2 -> If Action Subsystem3/Action
  Merge1/1 -> Angle_output/1

== system PMSM_FOC_Tractio/Motor_Control/Motor_Control_Funtion/Angle_Speed_100us/SMO/Delta_theta ==
  Est_theta : Inport
  Ealpha_est : Inport  Port=2
  Ebeta_est : Inport  Port=3
  Add : Sum
  Add1 : Sum
  Divide : Product  Inputs=*/
  Gain : Gain  Gain=-1
  Math Function : Math  Operator=magnitude^2  SignedPower=off  SaturateOnIntegerOverflow=on
  Math Function1 : Math  Operator=magnitude^2  SignedPower=off  SaturateOnIntegerOverflow=on
  Product : Product
  Product1 : Product
  Saturation : Saturate  UpperLimit=inf  LowerLimit=4.0
  Sine_Cosine : Subsystem  TreatAsAtomicUnit=on
      settings: RTWSystemCode=Nonreusable function  RTWFcnNameOpts=Use subsystem name
  Sqrt : Sqrt  SaturateOnIntegerOverflow=on
  delta_theta : Outport
  unit : Outport  Port=2
  wires:
  Est_theta/1 -> Sine_Cosine/1(P)
  Ealpha_est/1 -> Math Function/1, Product/2
  Sine_Cosine/1(Sin) -> Product1/1
  Ebeta_est/1 -> Math Function1/1, Product1/2
  Product/1 -> Add/1
  Product1/1 -> Add/2
  Add/1 -> Gain/1
  Math Function/1 -> Add1/1
  Math Function1/1 -> Add1/2
  Add1/1 -> Sqrt/1
  Sqrt/1 -> Saturation/1
  Gain/1 -> Divide/1
  Saturation/1 -> unit/1, Divide/2
  Divide/1 -> delta_theta/1
  Sine_Cosine/2(Cos) -> Product/1

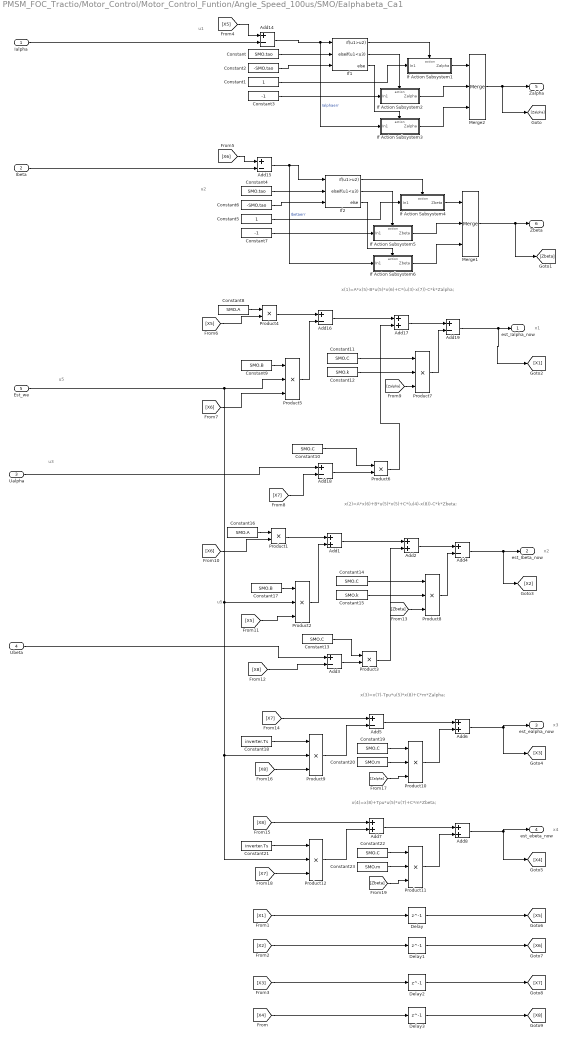
== system PMSM_FOC_Tractio/Motor_Control/Motor_Control_Funtion/Angle_Speed_100us/SMO/Ealphabeta_Ca1 ==
  note: x(4)=x(8)+Tpu*u(5)*x(7)+C*m*Zbeta;
  note: x(3)=x(7)-Tpu*u(5)*x(8)+C*m*Zalpha;
  note: x(2)=A*x(6)+B*u(5)*x(5)+C*(u(4)-x(8))-C*k*Zbeta;
  note: x(1)=A*x(5)-B*u(5)*x(6)+C*(u(3)-x(7))-C*k*Zalpha;
  note: x1
  note: u1
  note: u3
  note: u5
  note: u2
  note: u5
  note: x2
  note: x3
  note: x4
  Ialpha : Inport
  Ibeta : Inport  Port=2
  Ualpha : Inport  Port=3
  Ubeta : Inport  Port=4
  Est_we : Inport  Port=5
  Add{1..2,6..8,17} (6 alike) : Sum
  Add{3..5,14..16,18..19} (8 alike) : Sum  Inputs=+-
  Constant : Constant  Value=SMO.tao  OutDataTypeStr=single
  Constant1 : Constant  OutDataTypeStr=single
  Constant10 : Constant  Value=SMO.C  OutDataTypeStr=single
  Constant11 : Constant  Value=SMO.C  OutDataTypeStr=single
  Constant12 : Constant  Value=SMO.k  OutDataTypeStr=single
  Constant{13..14,19,22} (4 alike) : Constant  Value=SMO.C
  Constant15 : Constant  Value=SMO.k
  Constant16 : Constant  Value=SMO.A  OutDataTypeStr=single
  Constant17 : Constant  Value=SMO.B
  Constant18 : Constant  Value=inverter.Ts  OutDataTypeStr=single
  Constant2 : Constant  Value=-SMO.tao  OutDataTypeStr=single
  Constant20 : Constant  Value=SMO.m
  Constant21 : Constant  Value=inverter.Ts  OutDataTypeStr=single
  Constant23 : Constant  Value=SMO.m
  Constant3 : Constant  Value=-1  OutDataTypeStr=single
  Constant4 : Constant  Value=SMO.tao
  Constant5 : Constant  OutDataTypeStr=single
  Constant6 : Constant  Value=-SMO.tao
  Constant7 : Constant  Value=-1  OutDataTypeStr=single
  Constant8 : Constant  Value=SMO.A  OutDataTypeStr=single
  Constant9 : Constant  Value=SMO.B
  Delay{,1..3} (4 alike) : Delay  DelayLength=1  InitialCondition=0
  If Action Subsystem1 : Subsystem  TreatAsAtomicUnit=on
  If Action Subsystem2 : Subsystem  TreatAsAtomicUnit=on
  If Action Subsystem3 : Subsystem  TreatAsAtomicUnit=on
  If Action Subsystem4 : Subsystem  TreatAsAtomicUnit=on
  If Action Subsystem5 : Subsystem  TreatAsAtomicUnit=on
  If Action Subsystem6 : Subsystem  TreatAsAtomicUnit=on
  If1 : If  NumInputs=3  IfExpression=u1>u2  ElseIfExpressions=u1<u3
  If2 : If  NumInputs=3  IfExpression=u1>u2  ElseIfExpressions=u1<u3
  Merge1 : Merge  Inputs=3
  Merge2 : Merge  Inputs=3
  Product{1,3..4,6} (4 alike) : Product
  Product{2,5,7..12} (8 alike) : Product  Inputs=3
  est_Ialpha_now : Outport
  est_Ibeta_now : Outport  Port=2
  est_ealpha_now : Outport  Port=3
  est_ebeta_now : Outport  Port=4
  Zalpha : Outport  Port=5
  Zbeta : Outport  Port=6
  wires:
  Ialpha/1 -> Add14/2
  Add14/1 -> If Action Subsystem3/1(In1), If1/1  "Ialphaerr"
  Constant/1 -> If1/2
  If1/1 -> If Action Subsystem1/Action
  Constant1/1 -> If Action Subsystem1/1(In1)
  Constant3/1 -> If Action Subsystem2/1(In1)
  Constant2/1 -> If1/3
  If1/2 -> If Action Subsystem2/Action
  If1/3 -> If Action Subsystem3/Action
  If Action Subsystem1/1(Zalpha) -> Merge2/1
  If Action Subsystem2/1(Zalpha) -> Merge2/2
  If Action Subsystem3/1(Zalpha) -> Merge2/3
  Ibeta/1 -> Add15/2
  If2/1 -> If Action Subsystem4/Action
  If2/3 -> If Action Subsystem6/Action
  If Action Subsystem4/1(Zbeta) -> Merge1/1
  Constant5/1 -> If Action Subsystem4/1(In1)
  If2/2 -> If Action Subsystem5/Action
  Constant6/1 -> If2/3
  If Action Subsystem6/1(Zbeta) -> Merge1/3
  Constant7/1 -> If Action Subsystem5/1(In1)
  If Action Subsystem5/1(Zbeta) -> Merge1/2
  Add15/1 -> If2/1, If Action Subsystem6/1(In1)  "Ibetaerr"
  Constant4/1 -> If2/2
  Constant8/1 -> Product4/1
  Add19/1 -> [X1], est_Ialpha_now/1
  Product4/1 -> Add16/1
  Constant9/1 -> Product5/1
  Product5/1 -> Add16/2
  Add16/1 -> Add17/1
  Ualpha/1 -> Add18/1
  Add18/1 -> Product6/2
  Constant10/1 -> Product6/1
  Product6/1 -> Add17/2
  Add17/1 -> Add19/1
  Product7/1 -> Add19/2
  Constant11/1 -> Product7/1
  Constant12/1 -> Product7/2
  Product3/1 -> Add2/2
  Product8/1 -> Add4/2
  Constant15/1 -> Product8/2
  Constant16/1 -> Product1/1
  Add3/1 -> Product3/2
  Product2/1 -> Add1/2
  Add4/1 -> [X2], est_Ibeta_now/1
  Constant14/1 -> Product8/1
  Add1/1 -> Add2/1
  Constant13/1 -> Product3/1
  Ubeta/1 -> Add3/1
  Constant17/1 -> Product2/1
  Add2/1 -> Add4/1
  Product1/1 -> Add1/1
  Add6/1 -> est_ealpha_now/1, [X3]
  Constant18/1 -> Product9/1
  Product9/1 -> Add5/2
  Add5/1 -> Add6/1
  Constant19/1 -> Product10/1
  Constant20/1 -> Product10/2
  Product10/1 -> Add6/2
  Merge1/1 -> [Zbeta], Zbeta/1
  Constant21/1 -> Product12/1
  Constant22/1 -> Product11/1
  Est_we/1 -> Product12/2, Product9/2, Product2/2, Product5/2
  Product12/1 -> Add7/2
  Constant23/1 -> Product11/2
  Product11/1 -> Add8/2
  Add7/1 -> Add8/1
  Add8/1 -> [X4], est_ebeta_now/1
  Merge2/1 -> [Zalpha], Zalpha/1
  [X1] -> Delay/1
  [X2] -> Delay1/1
  [X3] -> Delay2/1
  [X4] -> Delay3/1
  Delay/1 -> [X5]
  Delay1/1 -> [X6]
  Delay2/1 -> [X7]
  Delay3/1 -> [X8]
  [X5] -> Add14/1
  [X6] -> Add15/1
  [X5] -> Product4/2
  [X6] -> Product5/3
  [X7] -> Add18/2
  [Zalpha] -> Product7/3
  [X6] -> Product1/2
  [X5] -> Product2/3
  [X8] -> Add3/2
  [Zbeta] -> Product8/3
  [X7] -> Add5/1
  [X8] -> Add7/1
  [X8] -> Product9/3
  [Zalpha] -> Product10/3
  [X7] -> Product12/3
  [Zbeta] -> Product11/3

== system PMSM_FOC_Tractio/Motor_Control/Motor_Control_Funtion/Angle_Speed_100us/SMO/PLL_PI ==
  in : Inport
  Add : Sum
  Discrete-Time Integrator : DiscreteIntegrator  SampleTime=Ts  ICPrevOutput=DiscIntNeverNeededParam  ICPrevScaledInput=DiscIntNeverNeededParam
  Gain2 : Gain  Gain=kp
  Gain3 : Gain  Gain=ki
  Saturation : Saturate  UpperLimit=inf  LowerLimit=-inf
  Scope : Scope  NumInputPorts=3
  Out : Outport
  wires:
  Gain2/1 -> Scope/1, Add/1
  Gain3/1 -> Discrete-Time Integrator/1
  Discrete-Time Integrator/1 -> Scope/2, Add/2
  in/1 -> Gain3/1, Gain2/1
  Add/1 -> Saturation/1
  Saturation/1 -> Scope/3, Out/1

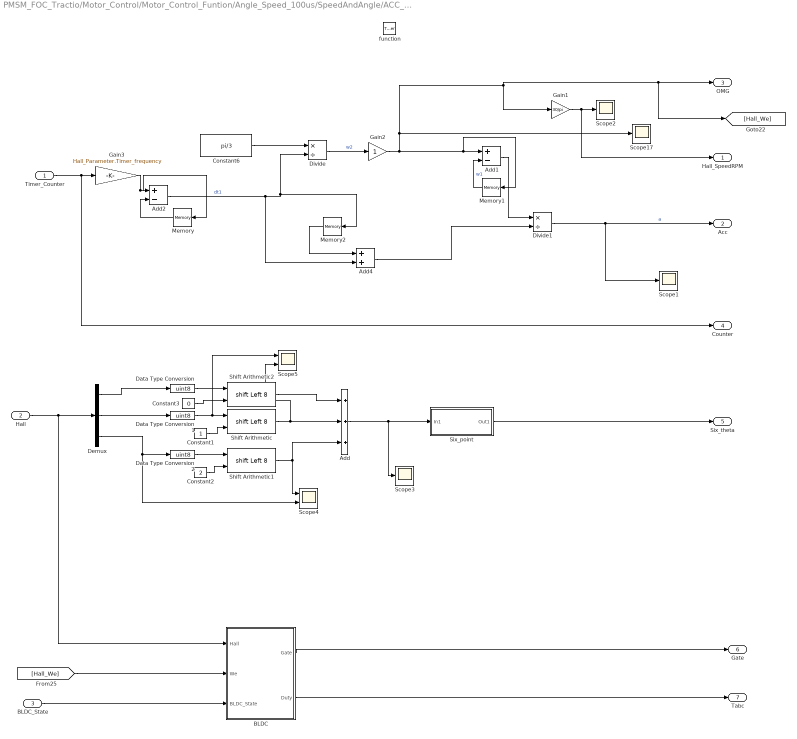
== system PMSM_FOC_Tractio/Motor_Control/Motor_Control_Funtion/Angle_Speed_100us/SpeedAndAngle/ACC_OMG ==
  Timer_Counter : Inport
  Hall : Inport  Port=2
  BLDC_State : Inport  Port=3
  function : TriggerPort  TriggerType=either  VariantControl=Variant
  Add : Sum  Inputs=+++
  Add1 : Sum  Inputs=+-
  Add2 : Sum  Inputs=+-
  Add4 : Sum
  BLDC : Subsystem
  Constant1 : Constant  OutDataTypeStr=uint8
  Constant2 : Constant  Value=2  OutDataTypeStr=uint8
  Constant3 : Constant  Value=0  OutDataTypeStr=uint8
  Constant6 : Constant  Value=pi/3  OutDataTypeStr=single
  Data Type Conversion : DataTypeConversion  OutDataTypeStr=uint8
  Data Type Conversion1 : DataTypeConversion  OutDataTypeStr=uint8
  Data Type Conversion2 : DataTypeConversion  OutDataTypeStr=uint8
  Demux : Demux  Outputs=3
  Divide : Product  Inputs=*/
  Divide1 : Product  Inputs=*/
  Gain1 : Gain  Gain=30/pi  OutDataTypeStr=Inherit: Same as input  ParamDataTypeStr=Inherit: Same as input
  Gain2 : Gain  OutDataTypeStr=Inherit: Same as input  ParamDataTypeStr=Inherit: Same as input
  Gain3 : Gain  Gain=Hall_Parameter.Timer_frequency
  Memory : Memory  InheritSampleTime=on
  Memory1 : Memory  InheritSampleTime=on
  Memory2 : Memory  InheritSampleTime=on
  Scope{1..3,17} (4 alike) : Scope
  Scope4 : Scope  NumInputPorts=2
  Scope5 : Scope  NumInputPorts=2
  Shift Arithmetic : ArithShift  BitShiftNumberSource=Input port  BitShiftNumber=8  BitShiftDirection=Left
      settings: InputPortMap=u0,p1
  Shift Arithmetic1 : ArithShift  BitShiftNumberSource=Input port  BitShiftNumber=8  BitShiftDirection=Left
      settings: InputPortMap=u0,p1
  Shift Arithmetic2 : ArithShift  BitShiftNumberSource=Input port  BitShiftNumber=8  BitShiftDirection=Left
      settings: InputPortMap=u0,p1
  Six_point : Subsystem  TreatAsAtomicUnit=on
  Hall_SpeedRPM : Outport
  Acc : Outport  Port=2
  OMG : Outport  Port=3
  Counter : Outport  Port=4
  Six_theta : Outport  Port=5
  Gate : Outport  Port=6  VectorParamsAs1DForOutWhenUnconnected=off
  Tabc : Outport  Port=7  VectorParamsAs1DForOutWhenUnconnected=off
  wires:
  Timer_Counter/1 -> Counter/1, Gain3/1
  Constant6/1 -> Divide/1
  Divide/1 -> Gain2/1  "w2"
  Memory/1 -> Add2/2
  Add2/1 -> Add4/2, Memory2/1, Divide/2  "dt1"
  Memory1/1 -> Add1/2  "w1"
  Add1/1 -> Divide1/1
  Add4/1 -> Divide1/2
  Divide1/1 -> Acc/1, Scope1/1  "a"
  Gain3/1 -> Memory/1, Add2/1
  Gain1/1 -> Hall_SpeedRPM/1, Scope2/1
  Memory2/1 -> Add4/1
  Demux/3 -> Scope4/2, Data Type Conversion2/1
  Data Type Conversion2/1 -> Shift Arithmetic1/1
  Constant2/1 -> Shift Arithmetic1/2
  Constant1/1 -> Shift Arithmetic/2
  Data Type Conversion1/1 -> Scope5/1, Shift Arithmetic/1
  Demux/1 -> Data Type Conversion/1
  Shift Arithmetic/1 -> Add/2, Scope5/2
  Demux/2 -> Data Type Conversion1/1
  Six_point/1(Out1) -> Six_theta/1
  Gain2/1 -> Gain1/1, [Hall_We], OMG/1, Scope17/1, Memory1/1, Add1/1
  Shift Arithmetic1/1 -> Add/3, Scope4/1
  Add/1 -> Scope3/1, Six_point/1(In1)
  Data Type Conversion/1 -> Shift Arithmetic2/1
  Shift Arithmetic2/1 -> Add/1
  Constant3/1 -> Shift Arithmetic2/2
  Hall/1 -> BLDC/1(Hall), Demux/1
  [Hall_We] -> BLDC/2(We)
  BLDC/2(Duty) -> Tabc/1
  BLDC/1(Gate) -> Gate/1
  BLDC_State/1 -> BLDC/3(BLDC_State)

== system PMSM_FOC_Tractio/Motor_Control/Motor_Control_Funtion/Angle_Speed_100us/SpeedAndAngle/ADC_IRQ ==
  Counter_ADC_IRQ : Inport
  Acc : Inport  Port=2
  OMG : Inport  Port=3
  Counter_Hall_IRQ : Inport  Port=4
  Six_theta : Inport  Port=5
  Add6 : Sum  Inputs=+-
  Add7 : Sum
  Gain2 : Gain  Gain=Hall_Parameter.Timer_frequency
  Gain3 : Gain  Gain=Hall_Parameter.Timer_frequency
  Gain4 : Gain  Gain=0.5
  Gain5 : Gain
  HallAngle_calibration : Subsystem
      settings: RTWSystemCode=Nonreusable function  RTWFcnNameOpts=Use subsystem name
  Math Function1 : Math  Operator=magnitude^2  SignedPower=off  SaturateOnIntegerOverflow=on
  Minus2 : Sum
  Product1 : Product
  Product2 : Product
  Hall_Angle : Outport
  wires:
  Gain5/1 -> Minus2/2
  Gain3/1 -> Math Function1/1
  Product2/1 -> Gain4/1
  Counter_Hall_IRQ/1 -> Add6/2
  Gain4/1 -> Minus2/1
  Add6/1 -> Gain3/1, Product1/2
  Math Function1/1 -> Product2/2
  Product1/1 -> Gain2/1
  Gain2/1 -> Gain5/1
  Counter_ADC_IRQ/1 -> Add6/1
  OMG/1 -> Product1/1
  Add7/1 -> HallAngle_calibration/1(Angle_input)
  Minus2/1 -> Add7/1
  Six_theta/1 -> Add7/2
  HallAngle_calibration/1(Angle_output) -> Hall_Angle/1  "SMO_Angle"
  Acc/1 -> Product2/1

== system PMSM_FOC_Tractio/Motor_Control/Motor_Control_Funtion/Angle_Speed_100us/SpeedAndAngle/Subsystem ==
  BLDC_State : Inport
  Hall : Inport  Port=2
  If1 : If  IfExpression=u1 ==1  ElseIfExpressions=u1 ==2  ShowElse=off
  Merge : Merge
  Merge1 : Merge
  Subsystem : Subsystem
  Subsystem1 : Subsystem
  Gate : Outport  VectorParamsAs1DForOutWhenUnconnected=off
  Duty_Set : Outport  Port=2  VectorParamsAs1DForOutWhenUnconnected=off
  wires:
  BLDC_State/1 -> If1/1
  If1/1 -> Subsystem/Action
  If1/2 -> Subsystem1/Action
  Hall/1 -> Subsystem1/1(Hall)
  Subsystem/1(Gate) -> Merge/1
  Subsystem1/1(Gate) -> Merge/2
  Merge/1 -> Gate/1
  Subsystem/2(Duty_Set) -> Merge1/1
  Subsystem1/2(Duty_Set) -> Merge1/2
  Merge1/1 -> Duty_Set/1

== system PMSM_FOC_Tractio/Motor_Control/Motor_Control_Funtion/Angle_Speed_100us/SpeedAndAngle/Subsystem1 ==
  Lock_Gate : Inport
  Lock_Duty : Inport  Port=2
  Hall_Gate : Inport  Port=3
  Hall_Duty : Inport  Port=4
  BLDC_State : Inport  Port=5
  If1 : If  IfExpression=u1 ==1 | u1 ==2  ElseIfExpressions=u1==3  ShowElse=off
  Merge : Merge
  Merge1 : Merge
  Subsystem : Subsystem
  Subsystem1 : Subsystem
  Gate : Outport  VectorParamsAs1DForOutWhenUnconnected=off
  Tabc : Outport  Port=2  VectorParamsAs1DForOutWhenUnconnected=off
  wires:
  BLDC_State/1 -> If1/1
  If1/1 -> Subsystem/Action
  Lock_Gate/1 -> Subsystem/1(In1)
  Lock_Duty/1 -> Subsystem/2(In2)
  If1/2 -> Subsystem1/Action
  Hall_Gate/1 -> Subsystem1/1(In1)
  Hall_Duty/1 -> Subsystem1/2(In2)
  Subsystem/1(Out1) -> Merge/1
  Subsystem1/1(Out1) -> Merge/2
  Merge/1 -> Gate/1
  Merge1/1 -> Tabc/1
  Subsystem/2(Out2) -> Merge1/1
  Subsystem1/2(Out2) -> Merge1/2

== system PMSM_FOC_Tractio/Motor_Control/Motor_Control_Funtion/Angle_Speed_100us/Speed_Angle_Selector/Hall ==
  In1 : Inport
  In2 : Inport  Port=2
  Action Port : ActionPort  ActionPortLabel=if(u1==1)
  Out1 : Outport
  Out2 : Outport  Port=2
  wires:
  In1/1 -> Out1/1
  In2/1 -> Out2/1

== system PMSM_FOC_Tractio/Motor_Control/Motor_Control_Funtion/Angle_Speed_100us/Speed_Angle_Selector/Resolver_Dir ==
  In1 : Inport
  In2 : Inport  Port=2
  Action Port : ActionPort  ActionPortLabel=if(u1==1)
  Out1 : Outport
  Out2 : Outport  Port=2
  wires:
  In1/1 -> Out1/1
  In2/1 -> Out2/1

== system PMSM_FOC_Tractio/Motor_Control/Motor_Control_Funtion/Angle_Speed_100us/Speed_Angle_Selector/Resolver_PLL ==
  In1 : Inport
  In2 : Inport  Port=2
  Action Port : ActionPort  ActionPortLabel=if(u1==1)
  Out1 : Outport
  Out2 : Outport  Port=2
  wires:
  In1/1 -> Out1/1
  In2/1 -> Out2/1

== system PMSM_FOC_Tractio/Motor_Control/Motor_Control_Funtion/Angle_Speed_100us/Speed_Angle_Selector/Sensorless ==
  In1 : Inport
  In2 : Inport  Port=2
  Action Port : ActionPort  ActionPortLabel=if(u1==1)
  Out1 : Outport
  Out2 : Outport  Port=2
  wires:
  In1/1 -> Out1/1
  In2/1 -> Out2/1

== system PMSM_FOC_Tractio/Motor_Control/Motor_Control_Funtion/Angle_Speed_100us/Speed_Resolver/Speed_cacl ==
  position : Inport  OutMin=-4*pi  OutMax=4*pi
      settings: AttributesFormatString="------------------\\nMin =  %<OutMin>\\nMax =  %<OutMax>"
  Convert_to_Uint32 : DataTypeConversion  OutDataTypeStr=int32  RndMeth=Simplest
  Difference_Wrap : Sum  Inputs=+-  AccumDataTypeStr=int32  OutDataTypeStr=int32
  Difference_to_Single : DataTypeConversion  OutDataTypeStr=single
  LPF : DiscreteFilter  Numerator=[0 0.5]  Denominator=[1 -0.5]
  Position_Delay : Delay  DelayLength=1
  RPM_Gain : Gain  Gain=60/(2*pi*pmsm.PolePairs)  ParamDataTypeStr=single  OutDataTypeStr=single
      settings: AttributesFormatString=---------------------------------\n%<Gain>
  Scale_Input : Gain  Gain=((2^31) - 1)/(4*pi)  ParamDataTypeStr=single  OutDataTypeStr=single
      settings: AttributesFormatString=---------------------------------\n%<Gain>
  Scale_Output : Gain  Gain=pi/(2^31 -1)/(inverter.Ts)  ParamDataTypeStr=single  OutDataTypeStr=single
      settings: AttributesFormatString=---------------------------------\n%<Gain>
  Scope1 : Scope  NumInputPorts=2
  Scope7 : Scope  NumInputPorts=2
  Wrap_To_Pi : Gain  Gain=4  RndMeth=Simplest  OutDataTypeStr=Inherit: Same as input  ParamDataTypeStr=Inherit: Same as input
  Speed_RPM : Outport  VectorParamsAs1DForOutWhenUnconnected=off
  wires:
  position/1 -> Scale_Input/1  "position"
  Scale_Input/1 -> Convert_to_Uint32/1
  Difference_to_Single/1 -> Scope7/1, Scale_Output/1
  Wrap_To_Pi/1 -> Difference_Wrap/1, Position_Delay/1
  Scale_Output/1 -> RPM_Gain/1  "We"
  Position_Delay/1 -> Difference_Wrap/2
  Convert_to_Uint32/1 -> Wrap_To_Pi/1
  Difference_Wrap/1 -> Difference_to_Single/1
  RPM_Gain/1 -> Scope7/2, Scope1/2, LPF/1  "Speed_RPM"
  LPF/1 -> Scope1/1, Speed_RPM/1  "Speed_RPM_Filtered"

== system PMSM_FOC_Tractio/Motor_Control/Motor_Control_Funtion/Angle_Speed_100us/Startup_OPL/Subsystem ==
  OPL_Speed : Inport
  OPL_Torque : Inport  Port=2
  Smo_theta : Inport  Port=3
  Action Port : ActionPort  ActionPortLabel=if(u1==2)
  2pi2 : Constant  Value=2*pi  OutDataTypeStr=single
  Constant1 : Constant  Value=1/OPL_Param.Acc_Times
  DT1 : DataTypeConversion  OutDataTypeStr=single
  DT2 : DataTypeConversion  OutDataTypeStr=single
  Discrete-Time Integrator1 : DiscreteIntegrator  SampleTime=-1  ICPrevOutput=DiscIntNeverNeededParam  ICPrevScaledInput=DiscIntNeverNeededParam
  Discrete-Time Integrator2 : DiscreteIntegrator  SampleTime=-1  ICPrevOutput=DiscIntNeverNeededParam  ICPrevScaledInput=DiscIntNeverNeededParam
  Mod2 : Math  Operator=mod  SignedPower=off  SaturateOnIntegerOverflow=on
  Product : Product
  Scope : Scope
  Scope1 : Scope
  Scope2 : Scope
  Scope3 : Scope  NumInputPorts=2
  Subtract : Sum  Inputs=+-
  We : Gain  Gain=pmsm.PolePairs*2*pi/60  OutDataTypeStr=single  ParamDataTypeStr=Inherit: Same as input
  Force_Angle : Outport
  OPL_Torque_Com : Outport  Port=2
  Delta_theta : Outport  Port=3
  Force_Switch : Outport  Port=4
  wires:
  DT1/1 -> Force_Angle/1  "Force_Angle"
  OPL_Torque/1 -> DT2/1
  DT2/1 -> OPL_Torque_Com/1
  We/1 -> Discrete-Time Integrator1/1  "Delta_Theta"
  2pi2/1 -> Mod2/2
  Mod2/1 -> Scope1/1, DT1/1  "Theta"
  OPL_Speed/1 -> Product/1
  Constant1/1 -> Product/2
  Product/1 -> Discrete-Time Integrator2/1
  Discrete-Time Integrator2/1 -> Scope/1, We/1
  Smo_theta/1 -> Scope3/1, Subtract/1
  Subtract/1 -> Scope2/1, Delta_theta/1
  Discrete-Time Integrator1/1 -> Scope3/2, Subtract/2, Force_Switch/1, Mod2/1

== system PMSM_FOC_Tractio/Motor_Control/Motor_Control_Funtion/Angle_Speed_100us/Startup_OPL/Subsystem1 ==
  OPL_Torque : Inport
  Delta_theta : Inport  Port=2
  Force_RPM : Inport  Port=3
  Force_Switch : Inport  Port=4
  Action Port : ActionPort  ActionPortLabel=elseif(u1==3)
  2pi2 : Constant  Value=2*pi  OutDataTypeStr=single
  Constant1 : Constant  Value=1/OPL_Param.Revup_Times
  Constant2 : Constant  Value=1/OPL_Param.Revup_Times
  DT1 : DataTypeConversion  OutDataTypeStr=single
  DT2 : DataTypeConversion  OutDataTypeStr=single
  Discrete-Time Integrator1 : DiscreteIntegrator  SampleTime=-1  ICPrevOutput=DiscIntNeverNeededParam  ICPrevScaledInput=DiscIntNeverNeededParam
  Discrete-Time Integrator2 : DiscreteIntegrator  SampleTime=-1  ICPrevOutput=DiscIntNeverNeededParam  ICPrevScaledInput=DiscIntNeverNeededParam
  Discrete-Time Integrator3 : DiscreteIntegrator  SampleTime=-1  ICPrevOutput=DiscIntNeverNeededParam  ICPrevScaledInput=DiscIntNeverNeededParam
  Divide : Product  Inputs=*/
  Divide1 : Product  Inputs=*/
  Iq_Command : Constant  Value=OPL_Param.Current_ref/2  SampleTime=-1
  Mod2 : Math  Operator=mod  SignedPower=off  SaturateOnIntegerOverflow=on
  Subtract : Sum  Inputs=+++
  Subtract1 : Sum  Inputs=+-
  We : Gain  Gain=pmsm.PolePairs*2*pi/60  OutDataTypeStr=single  ParamDataTypeStr=Inherit: Same as input
  Force_Angle : Outport
  OPL_Torque_Com : Outport  Port=2
  Force_Angle1 : Outport  Port=3
  wires:
  DT2/1 -> OPL_Torque_Com/1
  Delta_theta/1 -> Divide/1
  Constant1/1 -> Divide/2
  Divide/1 -> Discrete-Time Integrator1/1
  Discrete-Time Integrator1/1 -> Subtract/1
  Force_RPM/1 -> We/1
  We/1 -> Discrete-Time Integrator2/1  "Delta_Theta"
  Force_Switch/1 -> Subtract/2
  Discrete-Time Integrator2/1 -> Subtract/3
  DT1/1 -> Force_Angle/1
  Subtract/1 -> Force_Angle1/1, Mod2/1
  Mod2/1 -> DT1/1  "Theta"
  2pi2/1 -> Mod2/2
  OPL_Torque/1 -> Subtract1/1
  Constant2/1 -> Divide1/2
  Iq_Command/1 -> Divide1/1
  Divide1/1 -> Discrete-Time Integrator3/1
  Discrete-Time Integrator3/1 -> Subtract1/2
  Subtract1/1 -> DT2/1

== system PMSM_FOC_Tractio/Motor_Control/Motor_Control_Funtion/Control_Command_2ms/Speed_PI/Speed_PI ==
  PI_input : Inport
  HFI_State : Inport  Port=2
  Motor_State : Inport  Port=3
  Action Port : ActionPort  ActionPortLabel=if((u1==1)&(u2==3)|(u1~=1))
  HFI_Enalble : Constant  Value=HFI.Func_Enable  OutDataTypeStr=uint8
  If1 : If  NumInputs=3  IfExpression=(u1==3)&(u2==1)  ElseIfExpressions=(u2==0) & ((u3~=2)&(u3~=3))  ShowElse=off
  Merge : Merge
  Speed_Control : Subsystem
  Speed_Control1 : Subsystem
  PI_out : Outport  VectorParamsAs1DForOutWhenUnconnected=off
  wires:
  PI_input/1 -> Speed_Control1/1(Err), Speed_Control/1(Err)
  HFI_State/1 -> If1/1
  If1/1 -> Speed_Control/Action
  HFI_Enalble/1 -> If1/2
  If1/2 -> Speed_Control1/Action
  Merge/1 -> PI_out/1
  Speed_Control/1(PI_Out) -> Merge/1
  Speed_Control1/1(PI_Out) -> Merge/2
  Motor_State/1 -> If1/3

== system PMSM_FOC_Tractio/Motor_Control/Motor_Control_Funtion/FOC_Control_100us/FOC/Angle_set ==
  Reso_angle : Inport
  HFI_angle : Inport  Port=2
  HFI_state : Inport  Port=3
  IPD_Angle : Inport  Port=4
  HFI_AngleEnable : Constant  Value=HFI.Angle_Enable  OutDataTypeStr=uint8
  If1 : If  IfExpression=u1 ==1
  Subsystem : Subsystem
  Subsystem1 : Subsystem
  Out1 : Outport
  Out2 : Outport  Port=2
  wires:
  HFI_AngleEnable/1 -> If1/1
  If1/1 -> Subsystem/Action
  HFI_angle/1 -> Subsystem/2(HFI_angle)
  If1/2 -> Subsystem1/Action
  Reso_angle/1 -> Subsystem1/1(Reso_angle)
  Subsystem/1(Out1) -> Out1/1
  Subsystem1/1(Out1) -> Out2/1
  HFI_state/1 -> Subsystem/1(HFI_state)
  IPD_Angle/1 -> Subsystem/3(IPD_Angle)

== system PMSM_FOC_Tractio/Motor_Control/Motor_Control_Funtion/FOC_Control_100us/FOC/Clarke_Transform ==
  Phase_CurrentABC : Inport  PortDimensions=3
  Clark1 : Subsystem  TreatAsAtomicUnit=on
  Scope : Scope  NumInputPorts=2
  IAlpha : Outport  VectorParamsAs1DForOutWhenUnconnected=off
  IBeta : Outport  Port=2  VectorParamsAs1DForOutWhenUnconnected=off
  wires:
  Clark1/1(Ialpha) -> IAlpha/1, Scope/1
  Clark1/2(Ibeta) -> IBeta/1, Scope/2
  Phase_CurrentABC/1 -> Clark1/1(Iabc)
